simulink model "AMDwithAudio"  (R2020b)
settings: Solver=VariableStepAuto  StartTime=0.0  StopTime=15.0  RelTol=1e-3
libraries: dspvision x2, commchan3 x1, audiosources x1, dspsnks4 x1, dsparch4 x1, simulink_extras x1
settings Model: Creator=gideon  LastModifiedBy=gideon

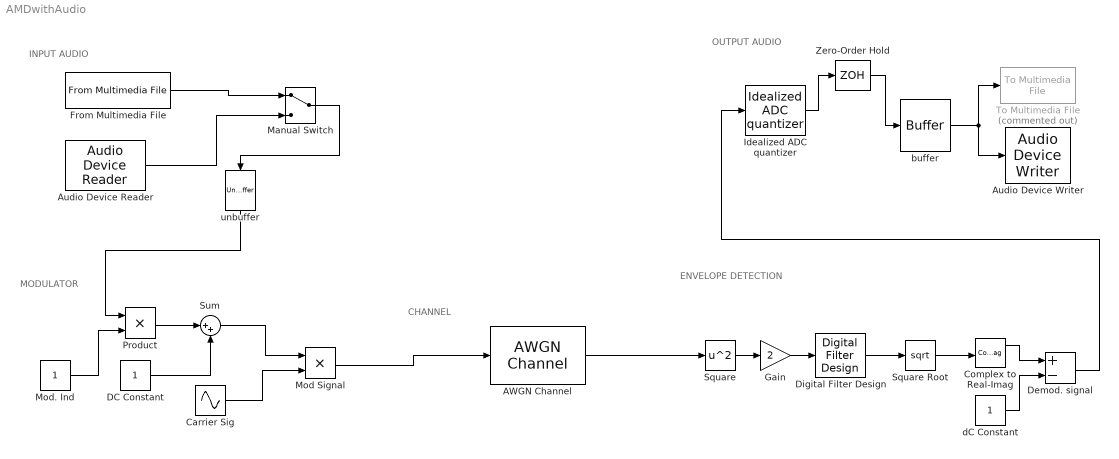
== system AMDwithAudio ==
  note: ENVELOPE DETECTION
  note: CHANNEL
  note: OUTPUT AUDIO
  note: MODULATOR
  note: INPUT AUDIO
  AWGN Channel : commchan3/AWGN Channel  InputProcessing=Columns as channels (frame based)  seed=1  noiseMode="Signal to noise ratio  (SNR)"  EbNodB=20  EsNodB=10  SNRdB=100  bitsPerSym=64  Ps=0.1  Tsym=1e-4  variance=1
  Audio Device Reader : audiosources/Audio Device Reader  Driver=CoreAudio  Device=MacBook Pro Microphone  SampleRate=48000  NumChannels=1  SamplesPerFrame=1024  BitDepth=16-bit integer  NumBuffers=10  DefaultInputChannelMapping=on  InputChannelMapping=1:2  OutputNumOverrunSamples=off  OutputDataType=double  DriverIdx=5  DeviceWarnFlag=''
      settings: SourceProductBaseCode=AU
  Audio Device Writer : dspsnks4/Audio Device Writer  Driver=CoreAudio  Device=MacBook Pro Speakers  InheritSampleRate=on  SampleRate=44100  BitDepth=24-bit integer  BufferSize=4096  NumBuffers=10  DefaultOutputChannelMapping=on  OutputChannelMapping=1:2  OutputNumUnderrunSamples=off  DriverIdx=5  DeviceWarnFlag=''
  Carrier Sig : Sin  Amplitude=1.5  Frequency=2*pi*8000  Phase=pi / 2  SampleTime=1/96000
  Complex to Real-Imag : ComplexToRealImag
  DC Constant : Constant
  Demod. signal : Sum  Inputs=+-
  Digital Filter Design : dsparch4/Digital Filter Design  mwdsp_browser_bugfix_var=off
  From Multimedia File : dspvision/From Multimedia File  inputFilename=/Users/gideon/MATLAB/projects/AMDSBwithAudio/merry.m4a  readRange=[1 Inf]  loop=on  numPlays=inf  outputStreams=Audio only  videoDataType=single  audioDataType=double  inheritSampleTime=on  userDefinedSampleTime=1/30  noAudioOutput=off  isIntensityVideo=off  fourcc=RGB  colorVideoFormat=Separate color signals  outputEOF=off  dataOrg=Column-major  audioFrameSize=1024  computeAudioFrameSize=off  outSamplingMode=Sample based
  Gain : Gain  Gain=2
  Idealized ADC quantizer : simulink_extras/Additional Discrete/Idealized ADC quantizer  NumberOfConverterBits=16  Vmin=0  Vmax=5  OutputDataType=int16  OutputNegativeValues=off
  Manual Switch : ManualSwitch
  Mod Signal : Product
  Mod. Ind : Constant
  Product : Product
  Square : Math  Operator=square  SaturateOnIntegerOverflow=on
  Square Root : Sqrt  OutputSignalType=complex  RndMeth=Round  SaturateOnIntegerOverflow=on
  Sum : Sum  Inputs=|++
  To Multimedia File : dspvision/To Multimedia File  Commented=on  outputFilename=/Users/gideon/Desktop/output.wav  streamSelection=Audio only  videoCompressor=None (uncompressed)  audioCompressor=None (uncompressed)  imagePorts=Separate color signals  fileType=WAV  audioDatatype=16-bit integer  fourcc=RGB  videoQuality=75  mj2000CompFactor=10
  Zero-Order Hold : ZeroOrderHold  SampleTime=1/96000
  buffer : Buffer  N=1024  OutputFrames=off
  dC Constant : Constant
  unbuffer : Unbuffer
  wires:
  DC Constant/1 -> Sum/2
  Zero-Order Hold/1 -> buffer/1
  Mod Signal/1 -> AWGN Channel/1
  dC Constant/1 -> Demod. signal/2
  buffer/1 -> Audio Device Writer/1, To Multimedia File/1
  Manual Switch/1 -> unbuffer/1
  AWGN Channel/1 -> Square/1
  Mod. Ind/1 -> Product/2
  Complex to Real-Imag/1 -> Demod. signal/1
  Product/1 -> Sum/1
  Carrier Sig/1 -> Mod Signal/2
  unbuffer/1 -> Product/1
  From Multimedia File/1 -> Manual Switch/1
  Gain/1 -> Digital Filter Design/1
  Idealized ADC quantizer/1 -> Zero-Order Hold/1
  Sum/1 -> Mod Signal/1
  Demod. signal/1 -> Idealized ADC quantizer/1
  Audio Device Reader/1 -> Manual Switch/2
  Square/1 -> Gain/1
  Digital Filter Design/1 -> Square Root/1
  Square Root/1 -> Complex to Real-Imag/1
